simulink model "Kalman_MPC"  (R2015a)
settings: Solver=ode4  StartTime=0.0  StopTime=20  FixedStep=0.01  RelTol=1e-3
settings Model: Creator=LAB425  LastModifiedBy=LAB425

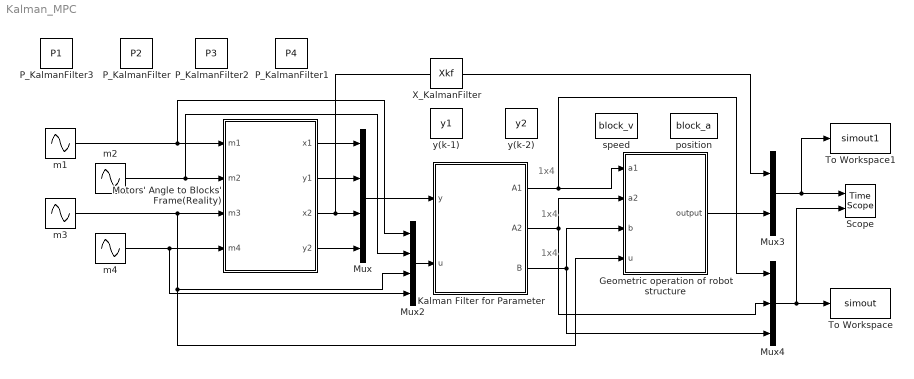
== system Kalman_MPC ==
  note: 1x4
  note: 1x4
  note: 1x4
  Geometric operation of robot structure : MATLAB Function  TreatAsAtomicUnit=on
  Kalman Filter for Parameter : MATLAB Function  TreatAsAtomicUnit=on
  "Motors' Angle to Blocks' Frame(Reality) " : MATLAB Function  TreatAsAtomicUnit=on
  Mux : Mux
  Mux2 : Mux
  Mux3 : Mux  Inputs=2
  Mux4 : Mux  Inputs=3
  P_KalmanFilter : DataStoreMemory  DataStoreName=P2  ReadBeforeWriteMsg=warning  WriteAfterWriteMsg=warning  WriteAfterReadMsg=warning  InitialValue=[0.001,0,0;0,0.002,0;0,0,0.001]  OutDataTypeStr=double
  P_KalmanFilter1 : DataStoreMemory  DataStoreName=P4  ReadBeforeWriteMsg=warning  WriteAfterWriteMsg=warning  WriteAfterReadMsg=warning  InitialValue=[0.001,0,0;0,0.002,0;0,0,0.001]  OutDataTypeStr=double
  P_KalmanFilter2 : DataStoreMemory  DataStoreName=P3  ReadBeforeWriteMsg=warning  WriteAfterWriteMsg=warning  WriteAfterReadMsg=warning  InitialValue=[0.001,0,0;0,0.002,0;0,0,0.001]  OutDataTypeStr=double
  P_KalmanFilter3 : DataStoreMemory  DataStoreName=P1  ReadBeforeWriteMsg=warning  WriteAfterWriteMsg=warning  WriteAfterReadMsg=warning  InitialValue=[0.001,0,0;0,0.002,0;0,0,0.001]  OutDataTypeStr=double
  Scope : TimeScope  NumInputPorts=2
  To Workspace : ToWorkspace  VariableName=simout  SaveFormat=Timeseries  SampleTime=-1
  To Workspace1 : ToWorkspace  VariableName=simout1  SaveFormat=Timeseries  SampleTime=-1
  X_KalmanFilter : DataStoreMemory  DataStoreName=Xkf  ReadBeforeWriteMsg=warning  WriteAfterWriteMsg=warning  WriteAfterReadMsg=warning  InitialValue=[0,0,0,0;0,0,0,0;0,0,0,0]  OutDataTypeStr=double
  m1 : Sin  SampleTime=0
  m2 : Sin  Frequency=2  SampleTime=0
  m3 : Sin  Phase=3.14  SampleTime=0
  m4 : Sin  Frequency=2  Phase=3.14  SampleTime=0
  position : DataStoreMemory  DataStoreName=block_a  ReadBeforeWriteMsg=warning  WriteAfterWriteMsg=warning  WriteAfterReadMsg=warning  OutDataTypeStr=double
  speed : DataStoreMemory  DataStoreName=block_v  ReadBeforeWriteMsg=warning  WriteAfterWriteMsg=warning  WriteAfterReadMsg=warning  OutDataTypeStr=double
  y(k-1) : DataStoreMemory  DataStoreName=y1  ReadBeforeWriteMsg=warning  WriteAfterWriteMsg=warning  WriteAfterReadMsg=warning  InitialValue=[0,0,0,0]  OutDataTypeStr=double
  y(k-2) : DataStoreMemory  DataStoreName=y2  ReadBeforeWriteMsg=warning  WriteAfterWriteMsg=warning  WriteAfterReadMsg=warning  InitialValue=[0,0,0,0]  OutDataTypeStr=double
  wires:
  m2/1 -> "Motors' Angle to Blocks' Frame(Reality) "/2(m2), Mux2/2
  m3/1 -> "Motors' Angle to Blocks' Frame(Reality) "/3(m3), Geometric operation of robot structure/4(u), Mux2/3
  m4/1 -> "Motors' Angle to Blocks' Frame(Reality) "/4(m4), Mux2/4
  "Motors' Angle to Blocks' Frame(Reality) "/2(y1) -> Mux/2
  "Motors' Angle to Blocks' Frame(Reality) "/3(x2) -> Mux3/1, Mux/3
  "Motors' Angle to Blocks' Frame(Reality) "/4(y2) -> Mux/4
  "Motors' Angle to Blocks' Frame(Reality) "/1(x1) -> Mux/1
  m1/1 -> Mux2/1, "Motors' Angle to Blocks' Frame(Reality) "/1(m1)
  Mux/1 -> Kalman Filter for Parameter/1(y)
  Mux2/1 -> Kalman Filter for Parameter/2(u)
  Kalman Filter for Parameter/1(A1) -> Mux4/1, Geometric operation of robot structure/1(a1)
  Kalman Filter for Parameter/2(A2) -> Mux4/2, Geometric operation of robot structure/2(a2)
  Kalman Filter for Parameter/3(B) -> Geometric operation of robot structure/3(b), Mux4/3
  Mux3/1 -> To Workspace1/1, Scope/1
  Geometric operation of robot structure/1(output) -> Mux3/2
  Mux4/1 -> Scope/2, To Workspace/1

== matlab function Kalman_MPC/Kalman Filter for Parameter ==
  data: y input; A1 output; u input; A2 output; B output; y1 data_store_memory; y2 data_store_memory; Xkf data_store_memory; P1 data_store_memory; P2 data_store_memory; P3 data_store_memory; P4 data_store_memory
function [A1,A2,B] = KalmanFilter(y,u)
global y1 y2 Xkf P1 P2 P3 P4
%% 单值参数识别（范例）
P = zeros(3,3,4);
P(:,:,1) = P1;
P(:,:,2) = P2;
P(:,:,3) = P3;
P(:,:,4) = P4;
Q = zeros(3,3);%过程噪声方差
R = 0.0000001;%测量噪声方差
F = 1;%状态转移矩阵
for i = 1:1:4
    H = [y1(i) y2(i) u(i)];%1x3
    Z = y(i) + sqrt(R) * randn(1);
    X_pre = F * Xkf(:,i);%3x1
    P_pre = F * P(:,:,i) * F' + Q;%3x3
    Kg = P_pre * H' * inv(H * P_pre * H' + R);%3x1
    Xkf(:,i) = X_pre + Kg * (Z - H * X_pre); %3x1
    P(:,:,i) = (eye(3,3) - Kg * H) * P_pre;
end
P1 = P(:,:,1);
P2 = P(:,:,2);
P3 = P(:,:,3);
P4 = P(:,:,4);

y2 = y1;
y1 = y;%[x1,y1,x2,y2]
A1 = Xkf(1,3);A2 = Xkf(2,3); B = Xkf(3,3);
%A1:a1的四个电机参数
%A2:a2的四个电机参数
%B:b的四个电机参数

== matlab function Kalman_MPC/Geometric operation of robot structure ==
  data: a1 input; a2 input; b input; output output; u input; block_v data_store_memory; block_a data_store_memory
function output = Robot(a1,a2,b,u)
global block_v block_a
%% 单电机状态方程
X = [0,1;-a2,-a1];
H = [0,b]';
C = [0,1];
delta_u = u - block_a;
v = delta_u / 0.01;
a = (v - block_v) / 0.01;
block_v = v;
block_a = u;
x = [v;a];
output = C * (X * x + H * u);
%%

== matlab function Kalman_MPC/Motors' Angle to Blocks' Frame(Reality)  ==
  data: x1 output; m1 input; y1 output; x2 output; m2 input; m3 input; m4 input; y2 output
function [x1,y1,x2,y2] = Signal(m1,m2,m3,m4)



%m1,m2,m3,m4为四个电机的当前时刻的角度值

%最远距离
D = 1.8;
% %螺距
% n = 0.02;
% %最大圈数
% ratio = D / n;
v=sqrt(0.01)*randn(4,1);
x1 = m1 * D + v(1);
y1 = m2 * D + v(2);
x2 = m3 * D + v(3);
y2 = m4 * D + v(4);
% x1 = m1 * D;
% y1 = m2 * D;
% x2 = m3 * D;
% y2 = m4 * D;

if x1>=2
    x1=2;
else
    if x1<=-2
        x1=-2;
    end
end
if x2>=2
    x2=2;
else
    if x2<=-2
        x2=-2;
    end
end
if y1>=2
    y1=2;
else
    if y1<=-2
        y1=-2;
    end
end
if y2>=2
    y2=2;
else
    if y2<=-2
        y2=-2;
    end
end
